simulink model "windmi_8"  (Simulink 6.6)
settings: Solver=ode15s  StartTime=0.0  StopTime=86400*3  RelTol=1e-4
values from neighbouring files (symbols this model uses):
  A = (L1*L-M^2)^(-1)    (= 0.000526438933084)    [windmi_setup.m]
  A_eff = WindmiCoeff(21)    [windmi_setup.m]
  alpha = WindmiCoeff(8)    [windmi_setup.m]
  B_tr = WindmiCoeff(20)    [windmi_setup.m]
  beta = WindmiCoeff(14)    [windmi_setup.m]
  C = WindmiCoeff(3)    [windmi_setup.m]
  C1 = WindmiCoeff(12)    [windmi_setup.m]
  Ic = 3.0e7    (= 30000000)    [windmi_setup.m]
  inv_dI = (del_I)^(-1)    (= 8e-06)    [windmi_setup.m]
  L = WindmiCoeff(1)    [windmi_setup.m]
  L1 = WindmiCoeff(11)    [windmi_setup.m]
  L2 = WindmiCoeff(18)    [windmi_setup.m]
  L_y = WindmiCoeff(22)    [windmi_setup.m]
  M = WindmiCoeff(2)    [windmi_setup.m]
  mu0 = WindmiCoeff(6)    [windmi_setup.m]
  Omega = WindmiCoeff(5)    [windmi_setup.m]
  R_A2 = WindmiCoeff(19)    [windmi_setup.m]
  R_prc = WindmiCoeff(16)    [windmi_setup.m]
  Sigma = WindmiCoeff(4)    [windmi_setup.m]
  SigmaI = WindmiCoeff(13)    [windmi_setup.m]
  tau_rc = WindmiCoeff(17)    [windmi_setup.m]
  tauE = WindmiCoeff(10)    [windmi_setup.m]
  taup = WindmiCoeff(9)    [windmi_setup.m]
undefined symbols (not defined in the file or in its folder): t_delay
settings Model: Creator=espencer  LastModifiedBy=ECE  ExtModeAutoUpdateStatusClock=off  TunableVars=A,A_eff,B_tr,C,C1,Ic,L,L1,L2,L_y,M,Omega,R_A2,R_prc,Sigma,SigmaI,alpha,alpha_F,beta,inv_dI,mu0,tauE,tau_rc,taup  TunableVarsStorageClass=Auto,Auto,Auto,Auto,Auto,Auto,Auto,Auto,Auto,Auto,Auto,Auto,Auto,Auto,Auto,Auto,Auto,Auto,Auto,Auto,Auto,Auto,Auto,Auto  TunableVarsTypeQualifier=,,,,,,,,,,,,,,,,,,,,,,,  BufferReuse=off
settings SolverCC: MaxConsecutiveZCs=10e6
settings DataIOCC: LimitDataPoints=off
settings OptimizationCC: BlockReduction=off  BooleanDataType=off  InlineParams=on  OptimizeBlockIOStorage=off  BufferReuse=off  ExpressionFolding=off  LocalBlockOutputs=off
settings DebuggingCC: SignalResolutionControl=TryResolveAllWithWarning  SolverPrmCheckMsg=none  MultiTaskDSMMsg=warning  MultiTaskCondExecSysMsg=none  StrictBusMsg=None
settings HardwareCC: TargetUnknown=on
settings RTWCC: IncludeERTFirstTime=on

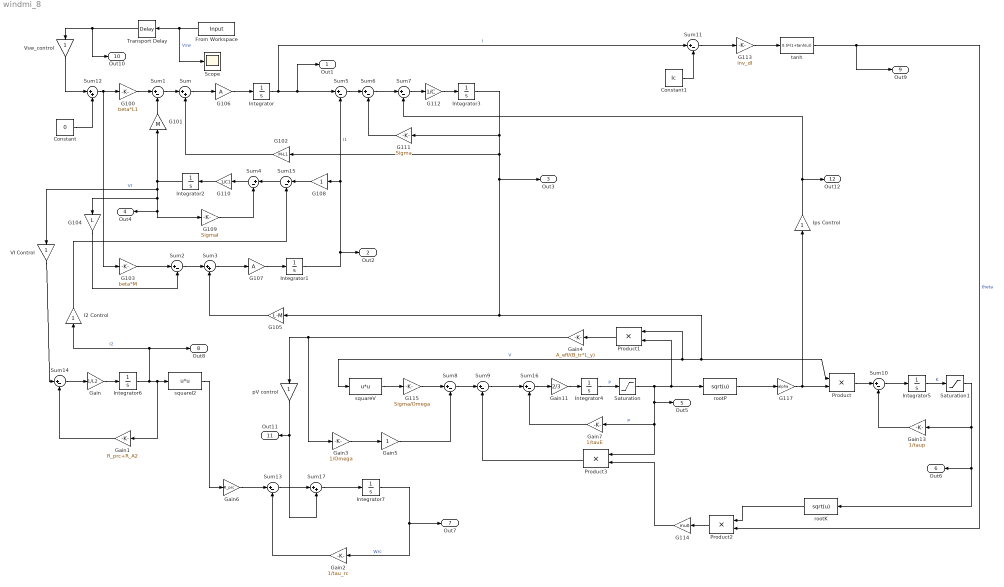
== system windmi_8 ==
  Constant : Constant  Value=0
  Constant1 : Constant  Value=Ic
  From Workspace : FromWorkspace  Orientation=left  VariableName=Input  SampleTime=0
  G100 : Gain  Gain=beta*L1  SaturateOnIntegerOverflow=on
  G101 : Gain  Orientation=up  Gain=M  SaturateOnIntegerOverflow=on
  G102 : Gain  Orientation=left  Gain=M-L1  SaturateOnIntegerOverflow=on
  G103 : Gain  Gain=beta*M  SaturateOnIntegerOverflow=on
  G104 : Gain  Orientation=down  Gain=L  SaturateOnIntegerOverflow=on
  G105 : Gain  Orientation=left  Gain=L-M  SaturateOnIntegerOverflow=on
  G106 : Gain  Gain=A  SaturateOnIntegerOverflow=on
  G107 : Gain  Gain=A  SaturateOnIntegerOverflow=on
  G108 : Gain  Orientation=left  SaturateOnIntegerOverflow=on
  G109 : Gain  Gain=SigmaI  SaturateOnIntegerOverflow=on
  G110 : Gain  Orientation=left  Gain=1/C1  SaturateOnIntegerOverflow=on
  G111 : Gain  Orientation=left  Gain=Sigma  SaturateOnIntegerOverflow=on
  G112 : Gain  Gain=1/C  SaturateOnIntegerOverflow=on
  G113 : Gain  Gain=inv_dI  SaturateOnIntegerOverflow=on
  G114 : Gain  Orientation=left  Gain=mu0  SaturateOnIntegerOverflow=on
  G115 : Gain  Gain=Sigma/Omega  SaturateOnIntegerOverflow=on
  G117 : Gain  Gain=alpha  SaturateOnIntegerOverflow=on
  Gain : Gain  Gain=1/L2  SaturateOnIntegerOverflow=on
  Gain1 : Gain  Orientation=left  Gain=R_prc+R_A2  SaturateOnIntegerOverflow=on
  Gain11 : Gain  Gain=2/3  SaturateOnIntegerOverflow=on
  Gain13 : Gain  Orientation=left  Gain=1/taup  SaturateOnIntegerOverflow=on
  Gain2 : Gain  Orientation=left  Gain=1/tau_rc  SaturateOnIntegerOverflow=on
  Gain3 : Gain  Gain=1/Omega  SaturateOnIntegerOverflow=on
  Gain4 : Gain  Orientation=left  Gain=A_eff/(B_tr*L_y)  SaturateOnIntegerOverflow=on
  Gain5 : Gain  SaturateOnIntegerOverflow=on
  Gain6 : Gain  Gain=R_prc  SaturateOnIntegerOverflow=on
  Gain7 : Gain  Orientation=left  Gain=1/tauE  SaturateOnIntegerOverflow=on
  I2 Control : Gain  Orientation=up  SaturateOnIntegerOverflow=on
  Integrator{,1,3..7} (7 alike) : Integrator
  Integrator2 : Integrator  Orientation=left
  Ips Control : Gain  Orientation=up  SaturateOnIntegerOverflow=on
  Product : Product  SaturateOnIntegerOverflow=on  RndMeth=Zero  InputSameDT=on
  Product1 : Product  Orientation=left  SaturateOnIntegerOverflow=on  RndMeth=Zero  InputSameDT=on
  Product2 : Product  Orientation=left  SaturateOnIntegerOverflow=on  RndMeth=Zero  InputSameDT=on
  Product3 : Product  Orientation=left  SaturateOnIntegerOverflow=on  RndMeth=Zero  InputSameDT=on
  Saturation : Saturate  UpperLimit=1  LowerLimit=1e-24
  Saturation1 : Saturate  UpperLimit=1e15  LowerLimit=1e-15
  Scope : Scope
  Sum{,3,12,17} (4 alike) : Sum  Inputs=|++  SaturateOnIntegerOverflow=on  InputSameDT=on
  Sum{1..2,5..11,13..14,16} (12 alike) : Sum  Inputs=|+-  SaturateOnIntegerOverflow=on  InputSameDT=on
  Sum15 : Sum  Orientation=left  Inputs=|+-  SaturateOnIntegerOverflow=on  InputSameDT=on
  Sum4 : Sum  Orientation=left  Inputs=|+-  SaturateOnIntegerOverflow=on  InputSameDT=on
  Transport Delay : TransportDelay  Orientation=left  DelayTime=t_delay  BufferSize=4096
  VI Control : Gain  Orientation=down  SaturateOnIntegerOverflow=on
  Vsw_control : Gain  Orientation=down  SaturateOnIntegerOverflow=on
  pV control : Gain  Orientation=down  SaturateOnIntegerOverflow=on
  rootK : Fcn  Orientation=left  Expr=sqrt(u)
  rootP : Fcn  Expr=sqrt(u)
  squareI2 : Fcn  Expr=u*u
  squareV : Fcn  Expr=u*u
  tanh : Fcn  Expr=0.5*(1+tanh(u))
  Out1 : Outport
  Out2 : Outport  Port=2
  Out3 : Outport  Port=3
  Out4 : Outport  Orientation=left  Port=4
  Out5 : Outport  Port=5
  Out6 : Outport  Orientation=left  Port=6
  Out7 : Outport  Port=7
  Out8 : Outport  Port=8
  Out9 : Outport  Port=9
  Out10 : Outport  Port=10
  Out11 : Outport  Orientation=left  Port=11
  Out12 : Outport  Port=12
  wires:
  Sum1/1 -> Sum/1
  G103/1 -> Sum2/1
  Sum2/1 -> Sum3/1
  Integrator2/1 -> G104/1, G109/1, Out4/1, VI Control/1, G101/1  "VI"
  G109/1 -> Sum4/2
  Integrator1/1 -> Out2/1, G108/1, Sum5/2  "I1"
  G101/1 -> Sum1/2
  G104/1 -> Sum2/2
  Integrator/1 -> Sum11/1, Sum5/1, Out1/1  "I"
  Sum5/1 -> Sum6/1
  Sum6/1 -> Sum7/1
  Sum7/1 -> G112/1
  G112/1 -> Integrator3/1
  Integrator3/1 -> G111/1, G102/1, Product/1, squareV/1, Product1/1, G105/1, Out3/1  "V"
  G111/1 -> Sum6/2
  G102/1 -> Sum/2
  G105/1 -> Sum3/2
  squareV/1 -> G115/1
  G115/1 -> Sum8/1
  Sum8/1 -> Sum9/1
  Gain11/1 -> Integrator4/1
  Integrator4/1 -> Saturation/1  "P"
  rootP/1 -> G117/1
  Sum10/1 -> Integrator5/1
  Gain13/1 -> Sum10/2
  Product/1 -> Sum10/1
  Constant1/1 -> Sum11/2
  Sum11/1 -> G113/1
  G113/1 -> tanh/1
  G106/1 -> Integrator/1
  Sum/1 -> G106/1
  G100/1 -> Sum1/1
  Sum3/1 -> G107/1
  G107/1 -> Integrator1/1
  Sum4/1 -> G110/1
  G110/1 -> Integrator2/1
  Ips Control/1 -> Sum7/2, Out12/1
  Sum12/1 -> G100/1, G103/1
  Product1/1 -> Gain4/1
  Sum14/1 -> Gain/1
  Gain/1 -> Integrator6/1
  Integrator6/1 -> Gain1/1, squareI2/1, I2 Control/1, Out8/1  "I2"
  Gain1/1 -> Sum14/2
  Sum15/1 -> Sum4/1
  G108/1 -> Sum15/1
  squareI2/1 -> Gain6/1
  Gain6/1 -> Sum13/1
  Sum13/1 -> Sum17/1
  Sum17/1 -> Integrator7/1
  Integrator7/1 -> Gain2/1, Out7/1  "Wrc"
  Gain2/1 -> Sum13/2
  Product3/1 -> Sum9/2
  tanh/1 -> Product2/2, Out9/1  "theta"
  G114/1 -> Product3/2
  Gain3/1 -> Gain5/1
  Gain5/1 -> Sum8/2
  Gain7/1 -> Sum16/2
  Sum9/1 -> Sum16/1
  Sum16/1 -> Gain11/1
  Gain4/1 -> Gain3/1, pV control/1
  I2 Control/1 -> Sum15/2
  VI Control/1 -> Sum14/1
  pV control/1 -> Sum17/2, Out11/1
  Product2/1 -> G114/1
  Constant/1 -> Sum12/2
  G117/1 -> Product/2, Ips Control/1
  rootK/1 -> Product2/1
  From Workspace/1 -> Transport Delay/1, Scope/1  "Vsw"
  Saturation/1 -> Product1/2, rootP/1, Product3/1, Gain7/1, Out5/1  "P"
  Integrator5/1 -> Saturation1/1  "K"
  Saturation1/1 -> Gain13/1, rootK/1, Out6/1
  Transport Delay/1 -> Vsw_control/1, Out10/1
  Vsw_control/1 -> Sum12/1
